simulink model "autopilot_with_kalman"  (R2019a)
settings: Solver=FixedStepAuto  StartTime=0.0  StopTime=200  FixedStep=0.01  RelTol=1e-3
values from neighbouring files (symbols this model uses):
  A = [ -0.322    0.052   0.028   -1.12   0.002 ... (first row only)    [A2_model.m]
  B = [ 0  0  0  0  7.5]'    [A2_model.m]
  C = [ 1 0 0 0 0 ... (first row only)    [A2_model.m]
  g = 9.81    [A2_model.m]
  k_d_phi = 0    [A2_Part1.m]    (also in A2_Part1_e.m = (2 * zeta_phi * omega_n_phi - a_phi_1)/a_phi_2)
  k_i_chi = 0    [A2_Part1.m]    (also in A2_Part1_e.m = omega_n_chi^2 * V_g/g)
  k_p_chi = 0    [A2_Part1.m]    (also in A2_Part1_e.m = 2 * zeta_chi * omega_n_chi * V_g/g)
  k_p_phi = 0    [A2_Part1.m]    (also in A2_Part1_e.m = delta_a_max/e_phi_max * sign(a_phi_2))
  V_g = V_a    [A2_Part1.m]    (also in A2_Part1_e.m)
libraries: simulink_extras x3, dspsrcs4 x2
settings Model: Creator=gustavoo  LastModifiedBy=gustavoo
settings DebuggingCC: ArithmeticOperatorsInVariantConditions=warning

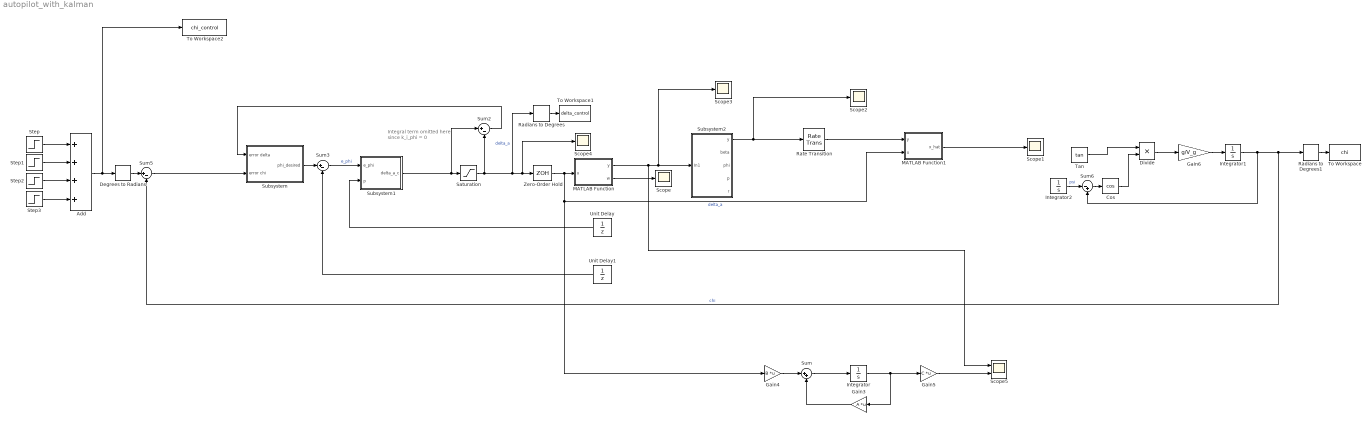
== system autopilot_with_kalman ==
  note: Integral term omitted here
      | since k_i_phi = 0
  Add : Sum  Inputs=++++
  Cos : Trigonometry  Operator=cos
  Degrees to Radians : simulink_extras/Transformations/Degrees to Radians
  Divide : Product  Inputs=**
  Gain3 : Gain  Gain=A  Multiplication=Matrix(K*u)
  Gain4 : Gain  Gain=B  Multiplication=Matrix(K*u)
  Gain5 : Gain  Gain=C  Multiplication=Matrix(K*u)
  Gain6 : Gain  Gain=g/V_g
  Integrator : Integrator
  Integrator1 : Integrator
  Integrator2 : Integrator
  MATLAB Function : MATLAB Function  TreatAsAtomicUnit=on
  MATLAB Function1 : MATLAB Function  TreatAsAtomicUnit=on
  Radians to Degrees : simulink_extras/Transformations/Radians to Degrees
  Radians to Degrees1 : simulink_extras/Transformations/Radians to Degrees
  Rate Transition : RateTransition
  Saturation : Saturate  UpperLimit=pi/6  LowerLimit=-pi/6
  Scope{,1..4} (5 alike) : Scope
  Scope5 : Scope  NumInputPorts=2
  Step : Step  Time=100  After=7.5  SampleTime=0
  Step1 : Step  Time=150  After=7.5  SampleTime=0
  Step2 : Step  Time=250  After=-15  SampleTime=0
  Step3 : Step  Time=300  After=0  SampleTime=0
  Subsystem : Subsystem
  Subsystem1 : Subsystem
  Subsystem2 : Subsystem
  Sum : Sum  Inputs=|++
  Sum2 : Sum  Inputs=|+-
  Sum3 : Sum  Inputs=|+-
  Sum5 : Sum  Inputs=|+-
  Sum6 : Sum  Inputs=|-+
  Tan : Trigonometry  Operator=tan
  To Workspace : ToWorkspace  VariableName=chi  SaveFormat=Timeseries  SampleTime=-1
  To Workspace1 : ToWorkspace  VariableName=delta_control  SaveFormat=Timeseries  SampleTime=-1
  To Workspace2 : ToWorkspace  VariableName=chi_control  SaveFormat=Timeseries  SampleTime=-1
  Unit Delay : UnitDelay  SampleTime=-1  HasFrameUpgradeWarning=on
  Unit Delay1 : UnitDelay  SampleTime=-1  HasFrameUpgradeWarning=on
  Zero-Order Hold : ZeroOrderHold  SampleTime=-1
  wires:
  Integrator1/1 -> Sum6/2, Sum5/2, Radians to Degrees1/1  "chi"
  Saturation/1 -> Scope4/1, Zero-Order Hold/1, Radians to Degrees/1, Sum2/2  "delta_a"
  Degrees to Radians/1 -> Sum5/1
  Step1/1 -> Add/2
  Step/1 -> Add/1
  Step3/1 -> Add/4
  Step2/1 -> Add/3
  Add/1 -> To Workspace2/1, Degrees to Radians/1
  Radians to Degrees1/1 -> To Workspace/1
  Radians to Degrees/1 -> To Workspace1/1
  Sum2/1 -> Subsystem/1(error delta)
  Gain6/1 -> Integrator1/1
  Divide/1 -> Gain6/1
  Integrator2/1 -> Sum6/1  "psi"
  Tan/1 -> Divide/1
  Sum6/1 -> Cos/1
  Cos/1 -> Divide/2
  Sum5/1 -> Subsystem/2(error chi)
  Subsystem/1(phi_desired) -> Sum3/1
  Subsystem1/1(delta_a_c) -> Sum2/1, Saturation/1
  Sum3/1 -> Subsystem1/1(e_phi)  "e_phi"
  MATLAB Function/2(w) -> Scope/1
  Unit Delay/1 -> Subsystem1/2(p)
  Unit Delay1/1 -> Sum3/2
  MATLAB Function/1(y) -> Scope5/1, Scope3/1, Subsystem2/1(In1)
  Subsystem2/1(y) -> Scope2/1, Rate Transition/1
  Rate Transition/1 -> MATLAB Function1/1(y)
  Gain4/1 -> Sum/1
  Zero-Order Hold/1 -> MATLAB Function1/2(u), Gain4/1, MATLAB Function/1(u)  "delta_a"
  Sum/1 -> Integrator/1
  Integrator/1 -> Gain3/1, Gain5/1
  Gain3/1 -> Sum/2
  Gain5/1 -> Scope5/2
  MATLAB Function1/1(x_hat) -> Scope1/1

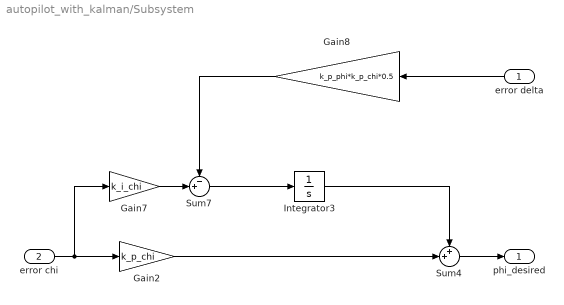
== system autopilot_with_kalman/Subsystem ==
  error delta : Inport
  error chi : Inport  Port=2
  Gain2 : Gain  Gain=k_p_chi
  Gain7 : Gain  Gain=k_i_chi
  Gain8 : Gain  Gain=k_p_phi*k_p_chi*0.5
  Integrator3 : Integrator
  Sum4 : Sum  Inputs=++|
  Sum7 : Sum  Inputs=-+|
  phi_desired : Outport
  wires:
  Gain8/1 -> Sum7/1
  Gain2/1 -> Sum4/2
  Integrator3/1 -> Sum4/1
  Gain7/1 -> Sum7/2
  error chi/1 -> Gain7/1, Gain2/1
  Sum7/1 -> Integrator3/1
  Sum4/1 -> phi_desired/1
  error delta/1 -> Gain8/1

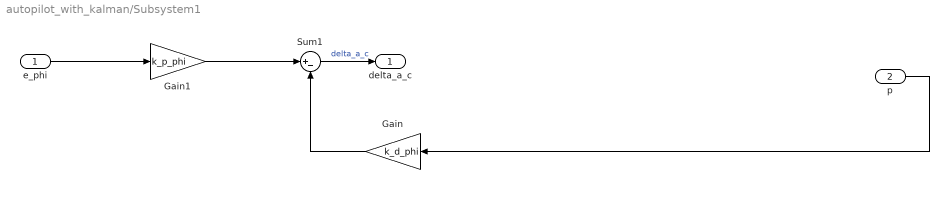
== system autopilot_with_kalman/Subsystem1 ==
  e_phi : Inport
  p : Inport  Port=2
  Gain : Gain  Gain=k_d_phi
  Gain1 : Gain  Gain=k_p_phi
  Sum1 : Sum  Inputs=|+-
  delta_a_c : Outport
  wires:
  Gain/1 -> Sum1/2
  Sum1/1 -> delta_a_c/1  "delta_a_c"
  Gain1/1 -> Sum1/1
  p/1 -> Gain/1
  e_phi/1 -> Gain1/1

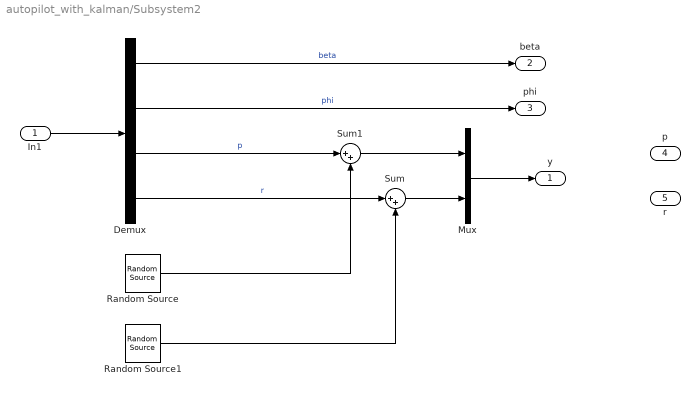
== system autopilot_with_kalman/Subsystem2 ==
  In1 : Inport
  Demux : Demux
  Mux : Mux  Inputs=2
  Random Source : dspsrcs4/Random Source  SrcType=Gaussian  NormMethod=Ziggurat  CltLength=12  MinVal=0  MaxVal=1  MeanVal=0  VarVal=0.2  RepMode=Not repeatable  rawSeed=1  IsInherit=off  SampMode=Discrete  SampTime=0.01  SampFrame=1  DataType=Double  OutComplex=Real  OutputFrames=off
  Random Source1 : dspsrcs4/Random Source  SrcType=Gaussian  NormMethod=Ziggurat  CltLength=12  MinVal=0  MaxVal=1  MeanVal=0  VarVal=0.2  RepMode=Not repeatable  rawSeed=1  IsInherit=off  SampMode=Discrete  SampTime=0.01  SampFrame=1  DataType=Double  OutComplex=Real  OutputFrames=off
  Sum : Sum  Inputs=|++
  Sum1 : Sum  Inputs=|++
  y : Outport
  beta : Outport  Port=2
  phi : Outport  Port=3
  p : Outport  Port=4
  r : Outport  Port=5
  wires:
  Demux/2 -> phi/1  "phi"
  In1/1 -> Demux/1
  Demux/1 -> beta/1  "beta"
  Demux/4 -> Sum/1  "r"
  Demux/3 -> Sum1/1  "p"
  Random Source/1 -> Sum1/2
  Random Source1/1 -> Sum/2
  Mux/1 -> y/1
  Sum1/1 -> Mux/1
  Sum/1 -> Mux/2

== matlab function autopilot_with_kalman/MATLAB Function1 ==
  data: y input; u input; x_hat output
function x_hat = fcn(y, u)
    persistent init_flag P_a_priori x_hat_a_priori P_post_priori y_a_priori S 

    if isempty(init_flag)
        S = load('kalman_variables');
        init_flag = 1;
        P_a_priori = S.P0_a_priori;
        x_hat_a_priori = S.x_hat_0_a_priori;
    end
    
    kalman_gain = P_a_priori*transpose(S.C)*inv(S.C*P_a_priori*transpose(S.C)+S.R);
    P_post_priori = P_a_priori - kalman_gain*S.C*P_a_priori - P_a_priori*transpose(S.C)...
        *transpose(kalman_gain) + kalman_gain*(S.C*P_a_priori*transpose(S.C)+S.R)*transpose(kalman_gain);
    y_a_priori = S.C*x_hat_a_priori;
    x_hat = x_hat_a_priori + kalman_gain*(y - y_a_priori);
    S.A_d
    x_hat
    x_hat_a_priori = S.A_d*x_hat + S.B_d*u;
    P_a_priori =  S.A_d*P_post_priori*transpose(S.A_d)+S.E_d*S.Q*transpose(S.E_d);
    
    end

== matlab function autopilot_with_kalman/MATLAB Function ==
  data: u input; y output; w output
function [y, w] = state_space(u)
% Generate the output of the state space

    % Persistent variables to be kept between function calls
    persistent counter; % Variable for checking if it is the first iteration.
    persistent x;       % The state x
    
   % The next line is necessary for generating unique process noise for every simulation.
   % Otherwise, the noise will be equal every time you run the simulation,
   % even though it is white. This has to do with how Matlab generates
   % random numbers. 
   coder.extrinsic('randn','rng');
    
    h = 0.01;       % Time step of Euler integration
    delta_a_c = u;  % Aileron input
    
    if isempty(counter)
      % First iteration
        counter = 1;
           
        % Initialize state space
        x = zeros(5,1);
        w = zeros(5,1); 
        rng('shuffle'); % Necessary for generating unique process noise for every simulation.
    
    else
        % State-space matrices
        A = [-0.322, 0.052, 0.028, -1.12, 0.002;
             0, 0, 1, -0.001, 0;
             -10.6, 0, -2.87, 0.46, -0.65;
             6.87, 0, -0.04, -0.32, -0.02;
             0, 0, 0, 0, -7.5];
 
        B = [0; 0; 0; 0; 7.5;];
        
        E = eye(5);
        
        % Discrete version
        Ad = eye(5) + h*A;
        Bd = h*B;
        Ed = E;
        
        % The Qd matrix in the assignment is given directly in discrete-time here and
        % therefore, it is not necessary to discretize E.
        Qd = h*10^-6*[0.001, 0, 0, 0, 0;
                  0, 1, 0, 0, 0;
                  0, 0, 100, 0, 0;
                  0, 0, 0, 10, 0;
                  0, 0, 0, 0, 0];
          
        w = sqrt(Qd)*randn(5,1,1); % The standard deviation must be multiplied with random numbers with a zero-mean unit variance random number to generate process noise. 
        
        % Discrete-time state space update
        x = Ad*x + Bd * delta_a_c + Ed*w;
    end
    y = x(1:4); % Return every state except the actuator state.
end
